simulink model "LCM"  (R2023a)
settings: Solver=FixedStepAuto  StartTime=0.0  StopTime=inf  RelTol=1e-3
settings Model: Creator=XboxX  LastModifiedBy=XboxX
settings OptimizationCC: OptimizeBlockIOStorage=off  OptimizeDataStoreBuffers=off  BusAssignmentInplaceUpdate=off
settings DebuggingCC: SFUnexpectedBacktrackingDiag=warning  SFNoUnconditionalDefaultTransitionDiag=warning  UnderSpecifiedDimensionMsg=warning
settings RTWCC: GenerateReport=on  BuildConfiguration=Debug  LaunchReport=on
settings CodeAppCC: ForceParamTrailComments=on  MATLABSourceComments=on  EnableCustomComments=on
settings GRTTargetCC: CombineSignalStateStructs=on  SupportVariableSizeSignals=on  MultiInstanceErrorCode=Warning

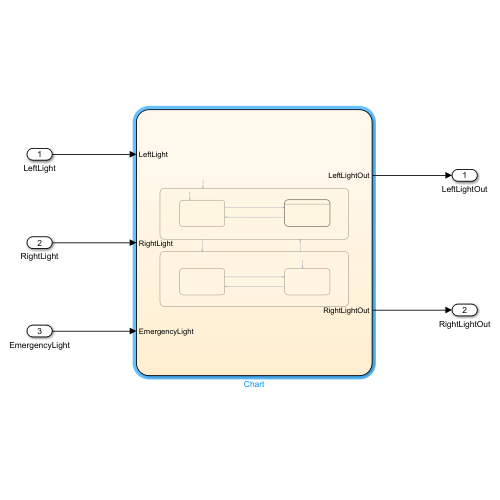
[thumbnail: Simulink's stored preview of the top-level diagram]
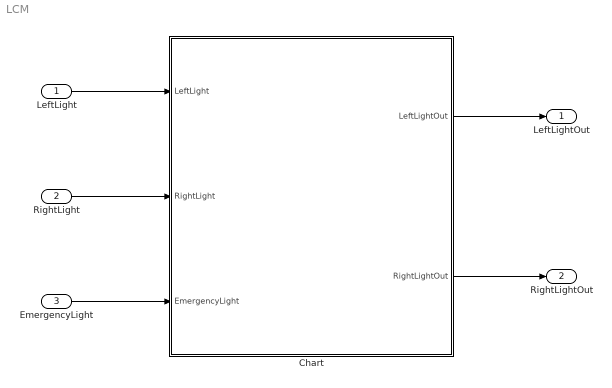
== system LCM ==
  LeftLight : Inport  OutDataTypeStr=boolean
  RightLight : Inport  Port=2  OutDataTypeStr=boolean
  EmergencyLight : Inport  Port=3  OutDataTypeStr=boolean
  Chart : Stateflow chart  TreatAsAtomicUnit=on
  LeftLightOut : Outport  OutDataTypeStr=boolean  PortDimensions=1
  RightLightOut : Outport  Port=2  OutDataTypeStr=boolean  PortDimensions=1
  wires:
  LeftLight/1 -> Chart/1(LeftLight)
  RightLight/1 -> Chart/2(RightLight)
  Chart/1(LeftLightOut) -> LeftLightOut/1
  Chart/2(RightLightOut) -> RightLightOut/1
  EmergencyLight/1 -> Chart/3(EmergencyLight)

== stateflow chart LCM/Chart ==
  state NORMAL
    state TURN
      state LEFT [parallel]
        settings: executionOrder=1
        state INACTIVE
          en:
          LeftLightOut = false;
        state ACTIVE
          state ON
            en:
            LeftLightOut = true;
          state OFF
            en:
            LeftLightOut = false;
          (default) -> NORMAL.TURN.LEFT.ACTIVE.ON
          NORMAL.TURN.LEFT.ACTIVE.ON -> NORMAL.TURN.LEFT.ACTIVE.OFF : [(true == after(50, tick))]
          NORMAL.TURN.LEFT.ACTIVE.OFF -> NORMAL.TURN.LEFT.ACTIVE.ON : [(true == after(50, tick))]
        (default) -> (junction 25)
        (junction 25) -> (junction 30) [order 1] : [(true == LeftLight)]
        (junction 30) -> NORMAL.TURN.LEFT.ACTIVE
        (junction 25) -> NORMAL.TURN.LEFT.INACTIVE [order 2]
        NORMAL.TURN.LEFT.INACTIVE -> NORMAL.TURN.LEFT.ACTIVE : [(true == LeftLight)]
        NORMAL.TURN.LEFT.ACTIVE -> NORMAL.TURN.LEFT.INACTIVE : [(false == LeftLight)]
      state RIGHT [parallel]
        settings: executionOrder=2
        state INACTIVE
          en:
          RightLightOut = false;
        state ACTIVE
          state ON
            en:
            RightLightOut = true;
          state OFF
            en:
            RightLightOut = false;
          (default) -> NORMAL.TURN.RIGHT.ACTIVE.ON
          NORMAL.TURN.RIGHT.ACTIVE.ON -> NORMAL.TURN.RIGHT.ACTIVE.OFF : [(true == after(50, tick))]
          NORMAL.TURN.RIGHT.ACTIVE.OFF -> NORMAL.TURN.RIGHT.ACTIVE.ON : [(true == after(50, tick))]
        (default) -> (junction 42)
        (junction 42) -> (junction 51) [order 1] : [(true == RightLight)]
        (junction 51) -> NORMAL.TURN.RIGHT.ACTIVE
        (junction 42) -> NORMAL.TURN.RIGHT.INACTIVE [order 2]
        NORMAL.TURN.RIGHT.INACTIVE -> NORMAL.TURN.RIGHT.ACTIVE : [(true == RightLight)]
        NORMAL.TURN.RIGHT.ACTIVE -> NORMAL.TURN.RIGHT.INACTIVE : [(false == RightLight)]
    state OFF
      en:
      LeftLightOut = false;
      RightLightOut = false;
    (default) -> NORMAL.OFF
    NORMAL.OFF -> TURN : [(true == LeftLight)...
        | || (true == RightLight)]
    TURN -> NORMAL.OFF : [(false == LeftLight)...
        | || (false == RightLight)]
  state EMERGENCY
    state OFF
      en:
      LeftLightOut = false;
      RightLightOut = false;
    state ON
      en:
      LeftLightOut = true;
      RightLightOut = true;
    (default) -> EMERGENCY.ON
    EMERGENCY.OFF -> EMERGENCY.ON : [(true == after(25,tick))]
    EMERGENCY.ON -> EMERGENCY.OFF : [(true == after(25,tick))]
  (default) -> NORMAL
  NORMAL -> EMERGENCY : [true == EmergencyLight]
  EMERGENCY -> NORMAL : [true ~= EmergencyLight]
  data: LeftLight input; RightLight input; LeftLightOut output; RightLightOut output; EmergencyLight input
